simulink model "sampleModel2432_pp_1_1_difftest"  (R2018a)
settings: Solver=VariableStepAuto  StartTime=0.0  StopTime=10.0  RelTol=1e-3
undefined symbols (not defined in the file or in its folder): DiscIntNeverNeededParam, sigbuilder_block
libraries: simulink x293
(part 2 of 7)

== system sampleModel2432_pp_1_1_difftest/cfblk201 ==
  cfblk1 : Inport
  cfblk11 : Inport  Port=2
  Action Port : ActionPort  ActionType=then
  cfblk{3,7..8,10} (4 alike) : DiscreteZeroPole  Poles=[0 0.5]  Gain=1  SampleTime=-1
  cfblk14 : Delay
  cfblk4 : simulink/Discrete/Difference  ICPrevInput=0.0  OutMin=[]  OutMax=[]  OutDataTypeStr=Inherit: Inherit via back propagation  OutDataType=fixdt(1, 16)  OutScaling=2^-10  DoSatur=off
  cfblk5 : simulink/Continuous/PID Controller  Controller=PID  TimeDomain=Discrete-time  SampleTime=-1  IntegratorMethod=Forward Euler  FilterMethod=Forward Euler  Form=Parallel  UseFilter=on  ControllerParametersSource=internal  P=1  I=1  D=0  N=100  InitialConditionSource=internal  InitialConditionForIntegrator=0  InitialConditionForFilter=0  ExternalReset=none  LimitOutput=off  UpperSaturationLimit=inf  LowerSaturationLimit=-inf  LinearizeAsGain=off  AntiWindupMode=none  Kb=1  TrackingMode=off  Kt=1  PParamMin=[]  PParamMax=[]  IParamMin=[]  IParamMax=[]  DParamMin=[]  DParamMax=[]  NParamMin=[]  NParamMax=[]  KbParamMin=[]  KbParamMax=[]  KtParamMin=[]  KtParamMax=[]  POutMin=[]  POutMax=[]  IOutMin=[]  IOutMax=[]  DOutMin=[]  DOutMax=[]  NOutMin=[]  NOutMax=[]  KbOutMin=[]  KbOutMax=[]  KtOutMin=[]  KtOutMax=[]  IntegratorOutMin=[]  IntegratorOutMax=[]  FilterOutMin=[]  FilterOutMax=[]  SumOutMin=[]  SumOutMax=[]  SumI1OutMin=[]  SumI1OutMax=[]  SumI2OutMin=[]  SumI2OutMax=[]  SumI3OutMin=[]  SumI3OutMax=[]  SumDOutMin=[]  SumDOutMax=[]  SaturationOutMin=[]  SaturationOutMax=[]  IntegratorContinuousStateAttributes=''  IntegratorStateMustResolveToSignalObject=off  IntegratorRTWStateStorageClass=Auto  FilterContinuousStateAttributes=''  FilterStateMustResolveToSignalObject=off  FilterRTWStateStorageClass=Auto  DifferentiatorICPrevScaledInput=0  DifferentiatorOutMin=[]  DifferentiatorOutMax=[]  FilterDiffOutCoefMin=[]  FilterDiffOutCoefMax=[]  SumDenOutMin=[]  SumDenOutMax=[]  SumNumOutMin=[]  SumNumOutMax=[]  ReciprocalOutMin=[]  ReciprocalOutMax=[]  DivideOutMin=[]  DivideOutMax=[]  TunerSelectOption=Transfer Function Based (PID Tuner App)
  cfblk6 : Delay
  cfblk9 : DiscreteFir
  cyemi_{218..226} (9 alike) : DataTypeConversion  OutDataTypeStr=double
  cfblk2 : Outport
  cfblk12 : Outport  Port=2
  cfblk13 : Outport  Port=3
  wires:
  cfblk1/1 -> cfblk2/1
  cfblk10/1 -> cfblk13/1
  cfblk7/1 -> cfblk12/1
  cfblk4/1 -> cyemi_218/1, cyemi_225/1
  cyemi_218/1 -> cfblk10/1
  cyemi_219/1 -> cfblk14/1
  cfblk6/1 -> cyemi_219/1
  cyemi_220/1 -> cfblk3/1
  cfblk8/1 -> cyemi_220/1
  cyemi_221/1 -> cfblk4/1
  cfblk11/1 -> cyemi_221/1
  cyemi_222/1 -> cfblk5/1
  cfblk14/1 -> cyemi_222/1
  cyemi_223/1 -> cfblk6/1
  cfblk5/1 -> cyemi_223/1
  cyemi_224/1 -> cfblk7/1
  cfblk9/1 -> cyemi_224/1
  cyemi_225/1 -> cfblk8/1
  cyemi_226/1 -> cfblk9/1
  cfblk3/1 -> cyemi_226/1

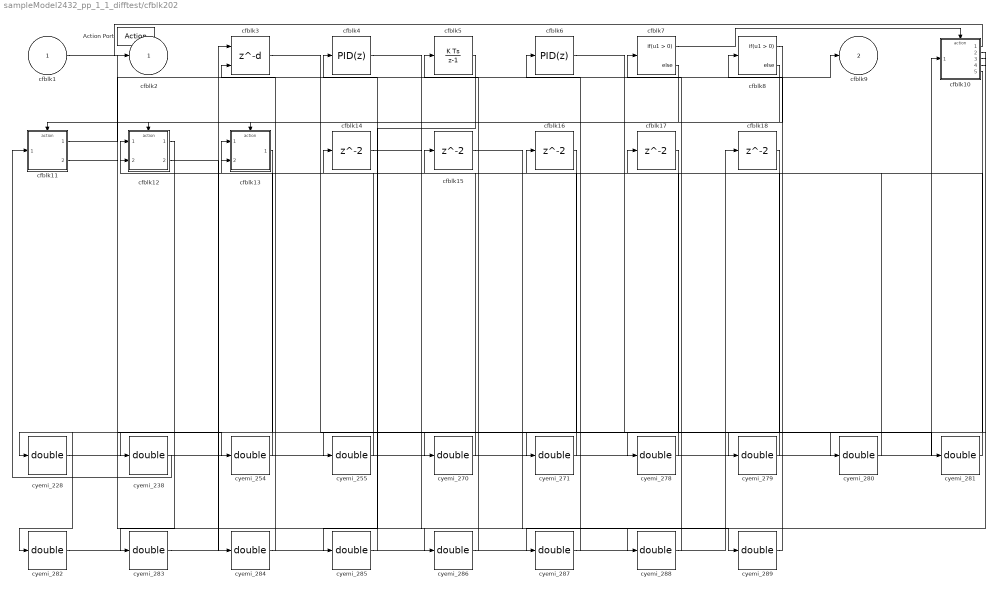
== system sampleModel2432_pp_1_1_difftest/cfblk202 ==
  cfblk1 : Inport
  Action Port : ActionPort  ActionType=else
  cfblk10 : Subsystem  TreatAsAtomicUnit=on
  cfblk11 : Subsystem  TreatAsAtomicUnit=on
  cfblk12 : Subsystem  TreatAsAtomicUnit=on
  cfblk13 : Subsystem  TreatAsAtomicUnit=on
  cfblk{14..18} (5 alike) : Delay
  cfblk3 : Delay  DelayLengthSource=Input port
      settings: InputPortMap=u0,p1
  cfblk4 : simulink/Continuous/PID Controller  Controller=PID  TimeDomain=Discrete-time  SampleTime=-1  IntegratorMethod=Forward Euler  FilterMethod=Forward Euler  Form=Parallel  UseFilter=on  ControllerParametersSource=internal  P=1  I=1  D=0  N=100  InitialConditionSource=internal  InitialConditionForIntegrator=0  InitialConditionForFilter=0  ExternalReset=none  LimitOutput=off  UpperSaturationLimit=inf  LowerSaturationLimit=-inf  LinearizeAsGain=off  AntiWindupMode=none  Kb=1  TrackingMode=off  Kt=1  PParamMin=[]  PParamMax=[]  IParamMin=[]  IParamMax=[]  DParamMin=[]  DParamMax=[]  NParamMin=[]  NParamMax=[]  KbParamMin=[]  KbParamMax=[]  KtParamMin=[]  KtParamMax=[]  POutMin=[]  POutMax=[]  IOutMin=[]  IOutMax=[]  DOutMin=[]  DOutMax=[]  NOutMin=[]  NOutMax=[]  KbOutMin=[]  KbOutMax=[]  KtOutMin=[]  KtOutMax=[]  IntegratorOutMin=[]  IntegratorOutMax=[]  FilterOutMin=[]  FilterOutMax=[]  SumOutMin=[]  SumOutMax=[]  SumI1OutMin=[]  SumI1OutMax=[]  SumI2OutMin=[]  SumI2OutMax=[]  SumI3OutMin=[]  SumI3OutMax=[]  SumDOutMin=[]  SumDOutMax=[]  SaturationOutMin=[]  SaturationOutMax=[]  IntegratorContinuousStateAttributes=''  IntegratorStateMustResolveToSignalObject=off  IntegratorRTWStateStorageClass=Auto  FilterContinuousStateAttributes=''  FilterStateMustResolveToSignalObject=off  FilterRTWStateStorageClass=Auto  DifferentiatorICPrevScaledInput=0  DifferentiatorOutMin=[]  DifferentiatorOutMax=[]  FilterDiffOutCoefMin=[]  FilterDiffOutCoefMax=[]  SumDenOutMin=[]  SumDenOutMax=[]  SumNumOutMin=[]  SumNumOutMax=[]  ReciprocalOutMin=[]  ReciprocalOutMax=[]  DivideOutMin=[]  DivideOutMax=[]  TunerSelectOption=Transfer Function Based (PID Tuner App)
  cfblk5 : DiscreteIntegrator  SampleTime=-1  ICPrevOutput=DiscIntNeverNeededParam  ICPrevScaledInput=DiscIntNeverNeededParam
  cfblk6 : simulink/Continuous/PID Controller  Controller=PID  TimeDomain=Discrete-time  SampleTime=-1  IntegratorMethod=Forward Euler  FilterMethod=Forward Euler  Form=Parallel  UseFilter=on  ControllerParametersSource=internal  P=1  I=1  D=0  N=100  InitialConditionSource=internal  InitialConditionForIntegrator=0  InitialConditionForFilter=0  ExternalReset=none  LimitOutput=off  UpperSaturationLimit=inf  LowerSaturationLimit=-inf  LinearizeAsGain=off  AntiWindupMode=none  Kb=1  TrackingMode=off  Kt=1  PParamMin=[]  PParamMax=[]  IParamMin=[]  IParamMax=[]  DParamMin=[]  DParamMax=[]  NParamMin=[]  NParamMax=[]  KbParamMin=[]  KbParamMax=[]  KtParamMin=[]  KtParamMax=[]  POutMin=[]  POutMax=[]  IOutMin=[]  IOutMax=[]  DOutMin=[]  DOutMax=[]  NOutMin=[]  NOutMax=[]  KbOutMin=[]  KbOutMax=[]  KtOutMin=[]  KtOutMax=[]  IntegratorOutMin=[]  IntegratorOutMax=[]  FilterOutMin=[]  FilterOutMax=[]  SumOutMin=[]  SumOutMax=[]  SumI1OutMin=[]  SumI1OutMax=[]  SumI2OutMin=[]  SumI2OutMax=[]  SumI3OutMin=[]  SumI3OutMax=[]  SumDOutMin=[]  SumDOutMax=[]  SaturationOutMin=[]  SaturationOutMax=[]  IntegratorContinuousStateAttributes=''  IntegratorStateMustResolveToSignalObject=off  IntegratorRTWStateStorageClass=Auto  FilterContinuousStateAttributes=''  FilterStateMustResolveToSignalObject=off  FilterRTWStateStorageClass=Auto  DifferentiatorICPrevScaledInput=0  DifferentiatorOutMin=[]  DifferentiatorOutMax=[]  FilterDiffOutCoefMin=[]  FilterDiffOutCoefMax=[]  SumDenOutMin=[]  SumDenOutMax=[]  SumNumOutMin=[]  SumNumOutMax=[]  ReciprocalOutMin=[]  ReciprocalOutMax=[]  DivideOutMin=[]  DivideOutMax=[]  TunerSelectOption=Transfer Function Based (PID Tuner App)
  cfblk7 : If  SampleTime=1
  cfblk8 : If  SampleTime=1
  cyemi_{228,238,254..255,270..271,278..289} (18 alike) : DataTypeConversion  OutDataTypeStr=double
  cfblk2 : Outport
  cfblk9 : Outport  Port=2
  wires:
  cfblk10/1(cfblk2) -> cfblk2/1
  cfblk11/1(cfblk2) -> cfblk9/1
  cfblk7/1 -> cfblk10/Action
  cfblk7/2 -> cfblk11/Action
  cfblk8/1 -> cfblk12/Action
  cfblk8/2 -> cfblk13/Action
  cyemi_228/1 -> cfblk10/1(cfblk1)
  cfblk13/1(cfblk2) -> cyemi_228/1
  cyemi_238/1 -> cfblk11/1(cfblk1)
  cfblk10/4(cfblk11) -> cyemi_238/1
  cyemi_254/1 -> cfblk12/1(cfblk1)
  cfblk1/1 -> cyemi_254/1
  cyemi_255/1 -> cfblk12/2(cfblk15)
  cfblk17/1 -> cyemi_255/1
  cyemi_270/1 -> cfblk13/1(cfblk1)
  cfblk18/1 -> cyemi_270/1
  cyemi_271/1 -> cfblk13/2(cfblk7)
  cfblk16/1 -> cyemi_271/1
  cyemi_278/1 -> cfblk14/1
  cfblk3/1 -> cyemi_278/1
  cyemi_279/1 -> cfblk15/1
  cfblk10/2(cfblk9) -> cyemi_279/1
  cyemi_280/1 -> cfblk16/1
  cfblk4/1 -> cyemi_280/1
  cyemi_281/1 -> cfblk17/1
  cfblk6/1 -> cyemi_281/1
  cyemi_282/1 -> cfblk18/1
  cfblk10/5(cfblk12) -> cyemi_282/1
  cyemi_283/1 -> cfblk3/1
  cfblk12/1(cfblk2) -> cyemi_283/1
  cyemi_284/1 -> cfblk3/2
  cfblk12/2(cfblk16) -> cyemi_284/1
  cyemi_285/1 -> cfblk4/1
  cfblk5/1 -> cyemi_285/1
  cyemi_286/1 -> cfblk5/1
  cfblk11/2(cfblk13) -> cyemi_286/1
  cyemi_287/1 -> cfblk6/1
  cfblk10/3(cfblk10) -> cyemi_287/1
  cyemi_288/1 -> cfblk7/1
  cfblk15/1 -> cyemi_288/1
  cyemi_289/1 -> cfblk8/1
  cfblk14/1 -> cyemi_289/1

== system sampleModel2432_pp_1_1_difftest/cfblk203 ==
  cfblk1 : Inport
  cfblk13 : Inport  Port=2
  cfblk14 : Inport  Port=3
  Action Port : ActionPort  ActionType=then
  cfblk3 : simulink/Continuous/PID Controller (2DOF)  Controller=PID  TimeDomain=Discrete-time  SampleTime=-1  IntegratorMethod=Forward Euler  FilterMethod=Forward Euler  Form=Parallel  UseFilter=on  ControllerParametersSource=internal  P=1  I=1  D=0  N=100  b=1  c=1  InitialConditionSource=internal  InitialConditionForIntegrator=0  InitialConditionForFilter=0  ExternalReset=none  LimitOutput=off  UpperSaturationLimit=inf  LowerSaturationLimit=-inf  LinearizeAsGain=off  AntiWindupMode=none  Kb=1  TrackingMode=off  Kt=1  PParamMin=[]  PParamMax=[]  IParamMin=[]  IParamMax=[]  DParamMin=[]  DParamMax=[]  NParamMin=[]  NParamMax=[]  bParamMin=[]  bParamMax=[]  cParamMin=[]  cParamMax=[]  KbParamMin=[]  KbParamMax=[]  KtParamMin=[]  KtParamMax=[]  POutMin=[]  POutMax=[]  IOutMin=[]  IOutMax=[]  DOutMin=[]  DOutMax=[]  NOutMin=[]  NOutMax=[]  bOutMin=[]  bOutMax=[]  cOutMin=[]  cOutMax=[]  KbOutMin=[]  KbOutMax=[]  KtOutMin=[]  KtOutMax=[]  IntegratorOutMin=[]  IntegratorOutMax=[]  FilterOutMin=[]  FilterOutMax=[]  SumOutMin=[]  SumOutMax=[]  Sum1OutMin=[]  Sum1OutMax=[]  Sum2OutMin=[]  Sum2OutMax=[]  Sum3OutMin=[]  Sum3OutMax=[]  SumI1OutMin=[]  SumI1OutMax=[]  SumI2OutMin=[]  SumI2OutMax=[]  SumI3OutMin=[]  SumI3OutMax=[]  SumDOutMin=[]  SumDOutMax=[]  SaturationOutMin=[]  SaturationOutMax=[]  IntegratorContinuousStateAttributes=''  IntegratorStateMustResolveToSignalObject=off  IntegratorRTWStateStorageClass=Auto  FilterContinuousStateAttributes=''  FilterStateMustResolveToSignalObject=off  FilterRTWStateStorageClass=Auto  DifferentiatorICPrevScaledInput=0  DifferentiatorOutMin=[]  DifferentiatorOutMax=[]  FilterDiffOutCoefMin=[]  FilterDiffOutCoefMax=[]  SumDenOutMin=[]  SumDenOutMax=[]  SumNumOutMin=[]  SumNumOutMax=[]  ReciprocalOutMin=[]  ReciprocalOutMax=[]  DivideOutMin=[]  DivideOutMax=[]  TunerSelectOption=Transfer Function Based (PID Tuner App)
  cfblk5 : Delay  ShowEnablePort=on
      settings: InputPortMap=u0,e6
  cfblk8 : DiscreteZeroPole  Poles=[0 0.5]  Gain=1  SampleTime=-1
  cyemi_{293..304} (12 alike) : DataTypeConversion  OutDataTypeStr=double
  cfblk2 : Outport
  cfblk15 : Outport  Port=2
  cfblk16 : Outport  Port=3
  wires:
  cfblk3/1 -> cfblk2/1
  cfblk14/1 -> cyemi_297/1, cyemi_304/1
  cfblk1/1 -> cyemi_294/1
  cfblk8/1 -> cyemi_295/1
  cyemi_296/1 -> cfblk3/1
  cyemi_297/1 -> cfblk3/2
  cyemi_299/1 -> cfblk5/1
  cyemi_300/1 -> cfblk5/2
  cfblk13/1 -> cyemi_300/1
  cfblk5/1 -> cyemi_301/1
  cyemi_303/1 -> cfblk8/1
  cyemi_304/1 -> cyemi_298/1
  cyemi_295/1 -> cfblk15/1
  cyemi_294/1 -> cyemi_302/1
  cyemi_301/1 -> cfblk16/1
  cyemi_302/1 -> cyemi_303/1, cyemi_296/1
  cyemi_298/1 -> cyemi_293/1
  cyemi_293/1 -> cyemi_299/1

== system sampleModel2432_pp_1_1_difftest/cfblk204 ==
  cfblk1 : Inport
  cfblk9 : Inport  Port=2
  cfblk10 : Inport  Port=3
  Action Port : ActionPort  ActionType=else
  cfblk13 : Subsystem  TreatAsAtomicUnit=on
  cfblk14 : Subsystem  TreatAsAtomicUnit=on
  cfblk15 : Delay
  cfblk16 : Delay
  cfblk3 : Delay
  cfblk4 : simulink/Discrete/Transfer Fcn Real Zero  ZeroZ=0.75  ICPrevInput=0.0  DoSatur=off
      settings: SourceProductName=Simulink  SourceProductBaseCode=SL
  cfblk5 : DiscreteFilter
  cfblk6 : DiscreteZeroPole  Poles=[0 0.5]  Gain=1  SampleTime=-1
  cfblk7 : DiscreteZeroPole  Poles=[0 0.5]  Gain=1  SampleTime=-1
  cfblk8 : If  SampleTime=1
  cyemi_{308..309,318..319,326..333} (12 alike) : DataTypeConversion  OutDataTypeStr=double
  cfblk2 : Outport
  cfblk11 : Outport  Port=2
  cfblk12 : Outport  Port=3
  wires:
  cfblk14/3(cfblk11) -> cfblk11/1
  cfblk14/4(cfblk12) -> cfblk12/1
  cfblk13/2(cfblk12) -> cfblk2/1
  cfblk8/1 -> cfblk13/Action
  cfblk8/2 -> cfblk14/Action
  cyemi_308/1 -> cfblk13/1(cfblk1)
  cfblk4/1 -> cyemi_308/1
  cyemi_309/1 -> cfblk13/2(cfblk11)
  cfblk14/2(cfblk10) -> cyemi_309/1
  cyemi_318/1 -> cfblk14/1(cfblk1)
  cfblk1/1 -> cyemi_318/1
  cyemi_319/1 -> cfblk14/2(cfblk9)
  cfblk15/1 -> cyemi_319/1
  cyemi_326/1 -> cfblk15/1
  cfblk3/1 -> cyemi_326/1
  cyemi_327/1 -> cfblk16/1
  cfblk13/1(cfblk2) -> cyemi_327/1
  cyemi_328/1 -> cfblk3/1
  cfblk5/1 -> cyemi_328/1
  cyemi_329/1 -> cfblk4/1
  cfblk7/1 -> cyemi_329/1
  cyemi_330/1 -> cfblk5/1
  cfblk14/1(cfblk2) -> cyemi_330/1
  cyemi_331/1 -> cfblk6/1
  cfblk10/1 -> cyemi_331/1
  cyemi_332/1 -> cfblk7/1
  cfblk6/1 -> cyemi_332/1
  cyemi_333/1 -> cfblk8/1
  cfblk16/1 -> cyemi_333/1

== system sampleModel2432_pp_1_1_difftest/cfblk205 ==
  cfblk1 : Inport
  Action Port : ActionPort  ActionType=then
  cfblk3 : simulink/Continuous/PID Controller  Controller=PID  TimeDomain=Discrete-time  SampleTime=-1  IntegratorMethod=Forward Euler  FilterMethod=Forward Euler  Form=Parallel  UseFilter=on  ControllerParametersSource=internal  P=1  I=1  D=0  N=100  InitialConditionSource=internal  InitialConditionForIntegrator=0  InitialConditionForFilter=0  ExternalReset=none  LimitOutput=off  UpperSaturationLimit=inf  LowerSaturationLimit=-inf  LinearizeAsGain=off  AntiWindupMode=none  Kb=1  TrackingMode=off  Kt=1  PParamMin=[]  PParamMax=[]  IParamMin=[]  IParamMax=[]  DParamMin=[]  DParamMax=[]  NParamMin=[]  NParamMax=[]  KbParamMin=[]  KbParamMax=[]  KtParamMin=[]  KtParamMax=[]  POutMin=[]  POutMax=[]  IOutMin=[]  IOutMax=[]  DOutMin=[]  DOutMax=[]  NOutMin=[]  NOutMax=[]  KbOutMin=[]  KbOutMax=[]  KtOutMin=[]  KtOutMax=[]  IntegratorOutMin=[]  IntegratorOutMax=[]  FilterOutMin=[]  FilterOutMax=[]  SumOutMin=[]  SumOutMax=[]  SumI1OutMin=[]  SumI1OutMax=[]  SumI2OutMin=[]  SumI2OutMax=[]  SumI3OutMin=[]  SumI3OutMax=[]  SumDOutMin=[]  SumDOutMax=[]  SaturationOutMin=[]  SaturationOutMax=[]  IntegratorContinuousStateAttributes=''  IntegratorStateMustResolveToSignalObject=off  IntegratorRTWStateStorageClass=Auto  FilterContinuousStateAttributes=''  FilterStateMustResolveToSignalObject=off  FilterRTWStateStorageClass=Auto  DifferentiatorICPrevScaledInput=0  DifferentiatorOutMin=[]  DifferentiatorOutMax=[]  FilterDiffOutCoefMin=[]  FilterDiffOutCoefMax=[]  SumDenOutMin=[]  SumDenOutMax=[]  SumNumOutMin=[]  SumNumOutMax=[]  ReciprocalOutMin=[]  ReciprocalOutMax=[]  DivideOutMin=[]  DivideOutMax=[]  TunerSelectOption=Transfer Function Based (PID Tuner App)
  cfblk4 : DiscreteFilter
  cfblk5 : simulink/Discrete/Transfer Fcn Real Zero  ZeroZ=0.75  ICPrevInput=0.0  DoSatur=off
      settings: SourceProductName=Simulink  SourceProductBaseCode=SL
  cfblk6 : simulink/Discrete/Transfer Fcn Real Zero  ZeroZ=0.75  ICPrevInput=0.0  DoSatur=off
      settings: SourceProductName=Simulink  SourceProductBaseCode=SL
  cyemi_{335..338} (4 alike) : DataTypeConversion  OutDataTypeStr=double
  cfblk2 : Outport
  cfblk7 : Outport  Port=2
  cfblk8 : Outport  Port=3
  wires:
  cfblk5/1 -> cyemi_335/1, cyemi_338/1
  cfblk3/1 -> cfblk2/1
  cfblk4/1 -> cfblk7/1, cfblk8/1
  cyemi_335/1 -> cfblk3/1
  cyemi_336/1 -> cfblk4/1
  cfblk6/1 -> cyemi_336/1
  cyemi_337/1 -> cfblk5/1
  cfblk1/1 -> cyemi_337/1
  cyemi_338/1 -> cfblk6/1

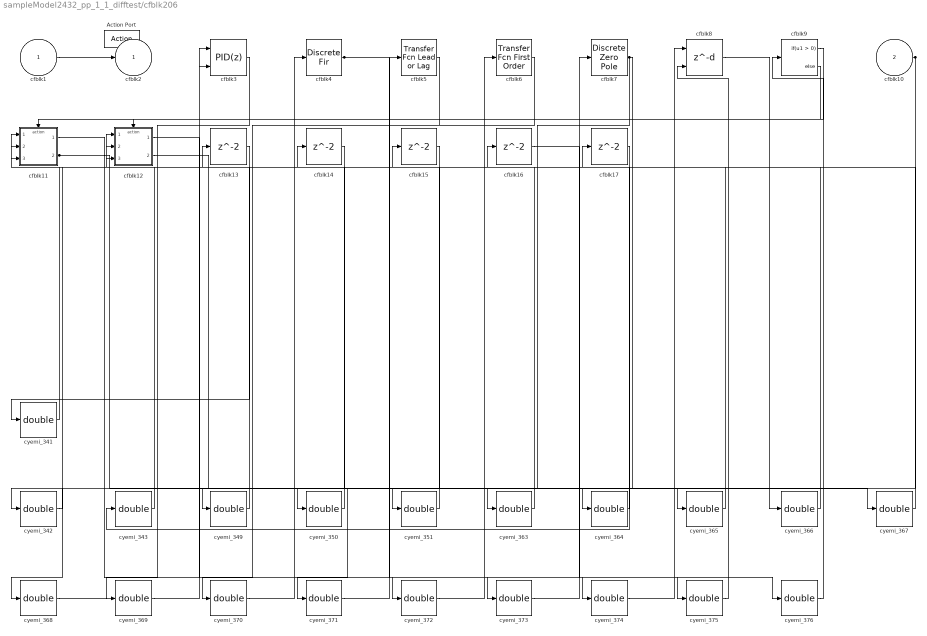
== system sampleModel2432_pp_1_1_difftest/cfblk206 ==
  cfblk1 : Inport
  cfblk10 : Inport  Port=2
  Action Port : ActionPort  ActionType=else
  cfblk11 : Subsystem  TreatAsAtomicUnit=on
  cfblk12 : Subsystem  TreatAsAtomicUnit=on
  cfblk{13..17} (5 alike) : Delay
  cfblk3 : simulink/Continuous/PID Controller (2DOF)  Controller=PID  TimeDomain=Discrete-time  SampleTime=-1  IntegratorMethod=Forward Euler  FilterMethod=Forward Euler  Form=Parallel  UseFilter=on  ControllerParametersSource=internal  P=1  I=1  D=0  N=100  b=1  c=1  InitialConditionSource=internal  InitialConditionForIntegrator=0  InitialConditionForFilter=0  ExternalReset=none  LimitOutput=off  UpperSaturationLimit=inf  LowerSaturationLimit=-inf  LinearizeAsGain=off  AntiWindupMode=none  Kb=1  TrackingMode=off  Kt=1  PParamMin=[]  PParamMax=[]  IParamMin=[]  IParamMax=[]  DParamMin=[]  DParamMax=[]  NParamMin=[]  NParamMax=[]  bParamMin=[]  bParamMax=[]  cParamMin=[]  cParamMax=[]  KbParamMin=[]  KbParamMax=[]  KtParamMin=[]  KtParamMax=[]  POutMin=[]  POutMax=[]  IOutMin=[]  IOutMax=[]  DOutMin=[]  DOutMax=[]  NOutMin=[]  NOutMax=[]  bOutMin=[]  bOutMax=[]  cOutMin=[]  cOutMax=[]  KbOutMin=[]  KbOutMax=[]  KtOutMin=[]  KtOutMax=[]  IntegratorOutMin=[]  IntegratorOutMax=[]  FilterOutMin=[]  FilterOutMax=[]  SumOutMin=[]  SumOutMax=[]  Sum1OutMin=[]  Sum1OutMax=[]  Sum2OutMin=[]  Sum2OutMax=[]  Sum3OutMin=[]  Sum3OutMax=[]  SumI1OutMin=[]  SumI1OutMax=[]  SumI2OutMin=[]  SumI2OutMax=[]  SumI3OutMin=[]  SumI3OutMax=[]  SumDOutMin=[]  SumDOutMax=[]  SaturationOutMin=[]  SaturationOutMax=[]  IntegratorContinuousStateAttributes=''  IntegratorStateMustResolveToSignalObject=off  IntegratorRTWStateStorageClass=Auto  FilterContinuousStateAttributes=''  FilterStateMustResolveToSignalObject=off  FilterRTWStateStorageClass=Auto  DifferentiatorICPrevScaledInput=0  DifferentiatorOutMin=[]  DifferentiatorOutMax=[]  FilterDiffOutCoefMin=[]  FilterDiffOutCoefMax=[]  SumDenOutMin=[]  SumDenOutMax=[]  SumNumOutMin=[]  SumNumOutMax=[]  ReciprocalOutMin=[]  ReciprocalOutMax=[]  DivideOutMin=[]  DivideOutMax=[]  TunerSelectOption=Transfer Function Based (PID Tuner App)
  cfblk4 : DiscreteFir
  cfblk5 : simulink/Discrete/Transfer Fcn Lead or Lag  PoleZ=0.95  ZeroZ=0.75  ICPrevOutput=0.0  ICPrevInput=0.0  DoSatur=off
      settings: SourceProductName=Simulink  SourceProductBaseCode=SL
  cfblk6 : simulink/Discrete/Transfer Fcn First Order  PoleZ=0.95  ICPrevOutput=0.0  DoSatur=off
      settings: SourceProductName=Simulink
  cfblk7 : DiscreteZeroPole  Poles=[0 0.5]  Gain=1  SampleTime=-1
  cfblk8 : Delay  DelayLengthSource=Input port
      settings: InputPortMap=u0,p1
  cfblk9 : If  SampleTime=1
  cyemi_{341..343,349..351,363..376} (20 alike) : DataTypeConversion  OutDataTypeStr=double
  cfblk2 : Outport
  wires:
  cfblk4/1 -> cyemi_365/1, cyemi_373/1
  cfblk1/1 -> cfblk2/1
  cfblk10/1 -> cyemi_368/1, cyemi_371/1
  cfblk7/1 -> cyemi_363/1, cyemi_364/1
  cfblk11/2(cfblk10) -> cyemi_350/1, cyemi_374/1
  cfblk9/1 -> cfblk11/Action
  cfblk9/2 -> cfblk12/Action
  cyemi_341/1 -> cfblk11/1(cfblk1)
  cfblk13/1 -> cyemi_341/1
  cyemi_342/1 -> cfblk11/2(cfblk8)
  cfblk3/1 -> cyemi_342/1
  cyemi_343/1 -> cfblk11/3(cfblk9)
  cfblk17/1 -> cyemi_343/1
  cyemi_349/1 -> cfblk12/1(cfblk1)
  cfblk5/1 -> cyemi_349/1
  cyemi_350/1 -> cfblk12/2(cfblk13)
  cyemi_351/1 -> cfblk12/3(cfblk14)
  cfblk15/1 -> cyemi_351/1
  cyemi_363/1 -> cfblk13/1
  cyemi_364/1 -> cfblk14/1
  cyemi_365/1 -> cfblk15/1
  cyemi_366/1 -> cfblk16/1
  cfblk8/1 -> cyemi_366/1
  cyemi_367/1 -> cfblk17/1
  cfblk12/2(cfblk15) -> cyemi_367/1
  cyemi_368/1 -> cfblk3/1
  cyemi_369/1 -> cfblk3/2
  cfblk14/1 -> cyemi_369/1
  cyemi_370/1 -> cfblk4/1
  cfblk6/1 -> cyemi_370/1
  cyemi_371/1 -> cfblk5/1
  cyemi_372/1 -> cfblk6/1
  cfblk11/1(cfblk2) -> cyemi_372/1
  cyemi_373/1 -> cfblk7/1
  cyemi_374/1 -> cfblk8/1
  cyemi_375/1 -> cfblk8/2
  cfblk12/1(cfblk2) -> cyemi_375/1
  cyemi_376/1 -> cfblk9/1
  cfblk16/1 -> cyemi_376/1

== system sampleModel2432_pp_1_1_difftest/cfblk207 ==
  cfblk1 : Inport
  cfblk8 : Inport  Port=2
  Action Port : ActionPort  ActionType=then
  cfblk10 : Delay
  cfblk4 : simulink/Discrete/Transfer Fcn Lead or Lag  PoleZ=0.95  ZeroZ=0.75  ICPrevOutput=0.0  ICPrevInput=0.0  DoSatur=off
      settings: SourceProductName=Simulink  SourceProductBaseCode=SL
  cfblk5 : DiscreteFir
  cfblk6 : Delay
  cfblk7 : Delay  ShowEnablePort=on
      settings: InputPortMap=u0,e6
  cyemi_{379..385} (7 alike) : DataTypeConversion  OutDataTypeStr=double
  cfblk2 : Outport
  cfblk9 : Outport  Port=2
  wires:
  cfblk1/1 -> cfblk9/1
  cyemi_379/1 -> cfblk10/1
  cfblk6/1 -> cyemi_379/1
  cfblk8/1 -> cyemi_380/1
  cyemi_381/1 -> cfblk4/1
  cfblk5/1 -> cyemi_381/1
  cyemi_382/1 -> cfblk5/1
  cyemi_383/1 -> cfblk6/1
  cfblk7/1 -> cyemi_383/1
  cyemi_384/1 -> cfblk7/1
  cfblk10/1 -> cyemi_384/1
  cyemi_385/1 -> cfblk7/2
  cfblk4/1 -> cyemi_385/1
  cyemi_380/1 -> cyemi_382/1, cfblk2/1

== system sampleModel2432_pp_1_1_difftest/cfblk208 ==
  cfblk1 : Inport
  Action Port : ActionPort  ActionType=else
  cfblk3 : Delay  ShowEnablePort=on
      settings: InputPortMap=u0,e6
  cfblk4 : DiscreteTransferFcn
  cfblk5 : simulink/Continuous/PID Controller  Controller=PID  TimeDomain=Discrete-time  SampleTime=-1  IntegratorMethod=Forward Euler  FilterMethod=Forward Euler  Form=Parallel  UseFilter=on  ControllerParametersSource=internal  P=1  I=1  D=0  N=100  InitialConditionSource=internal  InitialConditionForIntegrator=0  InitialConditionForFilter=0  ExternalReset=none  LimitOutput=off  UpperSaturationLimit=inf  LowerSaturationLimit=-inf  LinearizeAsGain=off  AntiWindupMode=none  Kb=1  TrackingMode=off  Kt=1  PParamMin=[]  PParamMax=[]  IParamMin=[]  IParamMax=[]  DParamMin=[]  DParamMax=[]  NParamMin=[]  NParamMax=[]  KbParamMin=[]  KbParamMax=[]  KtParamMin=[]  KtParamMax=[]  POutMin=[]  POutMax=[]  IOutMin=[]  IOutMax=[]  DOutMin=[]  DOutMax=[]  NOutMin=[]  NOutMax=[]  KbOutMin=[]  KbOutMax=[]  KtOutMin=[]  KtOutMax=[]  IntegratorOutMin=[]  IntegratorOutMax=[]  FilterOutMin=[]  FilterOutMax=[]  SumOutMin=[]  SumOutMax=[]  SumI1OutMin=[]  SumI1OutMax=[]  SumI2OutMin=[]  SumI2OutMax=[]  SumI3OutMin=[]  SumI3OutMax=[]  SumDOutMin=[]  SumDOutMax=[]  SaturationOutMin=[]  SaturationOutMax=[]  IntegratorContinuousStateAttributes=''  IntegratorStateMustResolveToSignalObject=off  IntegratorRTWStateStorageClass=Auto  FilterContinuousStateAttributes=''  FilterStateMustResolveToSignalObject=off  FilterRTWStateStorageClass=Auto  DifferentiatorICPrevScaledInput=0  DifferentiatorOutMin=[]  DifferentiatorOutMax=[]  FilterDiffOutCoefMin=[]  FilterDiffOutCoefMax=[]  SumDenOutMin=[]  SumDenOutMax=[]  SumNumOutMin=[]  SumNumOutMax=[]  ReciprocalOutMin=[]  ReciprocalOutMax=[]  DivideOutMin=[]  DivideOutMax=[]  TunerSelectOption=Transfer Function Based (PID Tuner App)
  cfblk6 : DiscreteFilter
  cfblk9 : Delay
  cyemi_{387..392} (6 alike) : DataTypeConversion  OutDataTypeStr=double
  cfblk2 : Outport
  cfblk7 : Outport  Port=2
  cfblk8 : Outport  Port=3
  wires:
  cfblk6/1 -> cfblk8/1
  cfblk4/1 -> cfblk7/1, cyemi_391/1
  cfblk5/1 -> cfblk2/1, cyemi_389/1, cyemi_392/1
  cyemi_387/1 -> cfblk3/1
  cfblk1/1 -> cyemi_387/1
  cyemi_388/1 -> cfblk3/2
  cfblk9/1 -> cyemi_388/1
  cyemi_389/1 -> cfblk4/1
  cyemi_390/1 -> cfblk5/1
  cfblk3/1 -> cyemi_390/1
  cyemi_391/1 -> cfblk6/1
  cyemi_392/1 -> cfblk9/1

== system sampleModel2432_pp_1_1_difftest/cfblk209 ==
  cfblk1 : Inport
  Action Port : ActionPort  ActionType=then
  cfblk3 : simulink/Discrete/Difference  ICPrevInput=0.0  OutMin=[]  OutMax=[]  OutDataTypeStr=Inherit: Inherit via back propagation  OutDataType=fixdt(1, 16)  OutScaling=2^-10  DoSatur=off
  cyemi_394 : DataTypeConversion  OutDataTypeStr=double
  cfblk2 : Outport
  cfblk4 : Outport  Port=2
  cfblk5 : Outport  Port=3
  cfblk6 : Outport  Port=4
  cfblk7 : Outport  Port=5
  wires:
  cfblk1/1 -> cfblk6/1, cfblk7/1, cyemi_394/1
  cfblk3/1 -> cfblk4/1, cfblk2/1, cfblk5/1
  cyemi_394/1 -> cfblk3/1

== system sampleModel2432_pp_1_1_difftest/cfblk210 ==
  cfblk1 : Inport
  Action Port : ActionPort  ActionType=else
  cfblk10 : Subsystem  TreatAsAtomicUnit=on
  cfblk11 : Subsystem  TreatAsAtomicUnit=on
  cfblk{12..15} (4 alike) : Delay
  cfblk3 : simulink/Discrete/Difference  ICPrevInput=0.0  OutMin=[]  OutMax=[]  OutDataTypeStr=Inherit: Inherit via back propagation  OutDataType=fixdt(1, 16)  OutScaling=2^-10  DoSatur=off
  cfblk4 : DiscreteFir
  cfblk5 : simulink/Discrete/Transfer Fcn Real Zero  ZeroZ=0.75  ICPrevInput=0.0  DoSatur=off
      settings: SourceProductName=Simulink  SourceProductBaseCode=SL
  cfblk6 : DiscreteStateSpace  SampleTime=-1
  cfblk7 : DiscreteIntegrator  SampleTime=-1  ICPrevOutput=DiscIntNeverNeededParam  ICPrevScaledInput=DiscIntNeverNeededParam
  cfblk8 : Delay  ShowEnablePort=on
      settings: InputPortMap=u0,e6
  cfblk9 : If  SampleTime=1
  cyemi_{398,405..406,420..431} (15 alike) : DataTypeConversion  OutDataTypeStr=double
  cfblk2 : Outport
  wires:
  cfblk11/3(cfblk14) -> cfblk2/1
  cfblk9/1 -> cfblk10/Action
  cfblk9/2 -> cfblk11/Action
  cyemi_398/1 -> cfblk10/1(cfblk1)
  cfblk13/1 -> cyemi_398/1
  cyemi_405/1 -> cfblk11/1(cfblk1)
  cfblk3/1 -> cyemi_405/1
  cyemi_406/1 -> cfblk11/2(cfblk12)
  cfblk15/1 -> cyemi_406/1
  cyemi_420/1 -> cfblk12/1
  cfblk10/1(cfblk2) -> cyemi_420/1
  cyemi_421/1 -> cfblk13/1
  cfblk5/1 -> cyemi_421/1
  cyemi_422/1 -> cfblk14/1
  cfblk8/1 -> cyemi_422/1
  cyemi_423/1 -> cfblk15/1
  cfblk7/1 -> cyemi_423/1
  cyemi_424/1 -> cfblk3/1
  cfblk1/1 -> cyemi_424/1
  cyemi_425/1 -> cfblk4/1
  cfblk6/1 -> cyemi_425/1
  cyemi_426/1 -> cfblk5/1
  cfblk10/2(cfblk7) -> cyemi_426/1
  cyemi_427/1 -> cfblk6/1
  cfblk11/1(cfblk2) -> cyemi_427/1
  cyemi_428/1 -> cfblk7/1
  cfblk11/2(cfblk13) -> cyemi_428/1
  cyemi_429/1 -> cfblk8/1
  cfblk12/1 -> cyemi_429/1
  cyemi_430/1 -> cfblk8/2
  cfblk4/1 -> cyemi_430/1
  cyemi_431/1 -> cfblk9/1
  cfblk14/1 -> cyemi_431/1

== system sampleModel2432_pp_1_1_difftest/cfblk211 ==
  cfblk1 : Inport
  cfblk7 : Inport  Port=2
  Action Port : ActionPort  ActionType=then
  cfblk5 : simulink/Discrete/Transfer Fcn Real Zero  ZeroZ=0.75  ICPrevInput=0.0  DoSatur=off
      settings: SourceProductName=Simulink  SourceProductBaseCode=SL
  cyemi_{434..437} (4 alike) : DataTypeConversion  OutDataTypeStr=double
  cfblk2 : Outport
  wires:
  cfblk5/1 -> cyemi_435/1
  cyemi_436/1 -> cfblk5/1
  cfblk7/1 -> cyemi_436/1
  cfblk1/1 -> cyemi_437/1
  cyemi_434/1 -> cfblk2/1
  cyemi_435/1 -> cyemi_434/1

== system sampleModel2432_pp_1_1_difftest/cfblk212 ==
  cfblk1 : Inport
  cfblk9 : Inport  Port=2
  Action Port : ActionPort  ActionType=else
  cfblk3 : DiscreteZeroPole  Poles=[0 0.5]  Gain=1  SampleTime=-1
  cfblk4 : DiscreteTransferFcn
  cfblk5 : DiscreteFilter
  cfblk6 : simulink/Discrete/Transfer Fcn Real Zero  ZeroZ=0.75  ICPrevInput=0.0  DoSatur=off
      settings: SourceProductName=Simulink  SourceProductBaseCode=SL
  cfblk7 : DiscreteIntegrator  SampleTime=-1  ICPrevOutput=DiscIntNeverNeededParam  ICPrevScaledInput=DiscIntNeverNeededParam
  cfblk8 : simulink/Discrete/Transfer Fcn First Order  PoleZ=0.95  ICPrevOutput=0.0  DoSatur=off
      settings: SourceProductName=Simulink
  cyemi_{440..445} (6 alike) : DataTypeConversion  OutDataTypeStr=double
  cfblk2 : Outport
  cfblk10 : Outport  Port=2
  cfblk11 : Outport  Port=3
  cfblk12 : Outport  Port=4
  wires:
  cfblk7/1 -> cfblk12/1, cyemi_441/1
  cfblk5/1 -> cfblk10/1, cyemi_443/1
  cfblk3/1 -> cfblk11/1
  cfblk4/1 -> cfblk2/1
  cyemi_440/1 -> cfblk3/1
  cfblk8/1 -> cyemi_440/1
  cyemi_441/1 -> cfblk4/1
  cyemi_442/1 -> cfblk5/1
  cfblk9/1 -> cyemi_442/1
  cyemi_443/1 -> cfblk6/1
  cyemi_444/1 -> cfblk7/1
  cfblk1/1 -> cyemi_444/1
  cyemi_445/1 -> cfblk8/1
  cfblk6/1 -> cyemi_445/1

== system sampleModel2432_pp_1_1_difftest/cfblk213 ==
  cfblk1 : Inport
  cfblk7 : Inport  Port=2
  cfblk8 : Inport  Port=3
  Action Port : ActionPort  ActionType=then
  cfblk3 : Delay
  cfblk5 : DiscreteIntegrator  SampleTime=-1  ICPrevOutput=DiscIntNeverNeededParam  ICPrevScaledInput=DiscIntNeverNeededParam
  cfblk6 : DiscreteZeroPole  Poles=[0 0.5]  Gain=1  SampleTime=-1
  cyemi_{449..452} (4 alike) : DataTypeConversion  OutDataTypeStr=double
  cfblk2 : Outport
  cfblk9 : Outport  Port=2
  wires:
  cfblk5/1 -> cfblk9/1
  cfblk3/1 -> cfblk2/1
  cyemi_449/1 -> cfblk3/1
  cfblk7/1 -> cyemi_450/1
  cyemi_451/1 -> cfblk5/1
  cfblk8/1 -> cyemi_451/1
  cyemi_452/1 -> cfblk6/1
  cfblk1/1 -> cyemi_452/1
  cyemi_450/1 -> cyemi_449/1

== system sampleModel2432_pp_1_1_difftest/cfblk214 ==
  cfblk1 : Inport
  cfblk9 : Inport  Port=2
  Action Port : ActionPort  ActionType=else
  cfblk10 : Delay
  cfblk3 : simulink/Discrete/Tapped Delay  vinit=0.0  samptime=-1  NumDelays=1  DelayOrder=Oldest  includeCurrent=off
  cfblk4 : simulink/Discrete/Tapped Delay  vinit=0.0  samptime=-1  NumDelays=1  DelayOrder=Oldest  includeCurrent=off
  cfblk5 : DiscreteFilter
  cfblk6 : simulink/Discrete/Transfer Fcn Real Zero  ZeroZ=0.75  ICPrevInput=0.0  DoSatur=off
      settings: SourceProductName=Simulink  SourceProductBaseCode=SL
  cfblk7 : DiscreteIntegrator  SampleTime=-1  ICPrevOutput=DiscIntNeverNeededParam  ICPrevScaledInput=DiscIntNeverNeededParam
  cfblk8 : simulink/Continuous/PID Controller  Controller=PID  TimeDomain=Discrete-time  SampleTime=-1  IntegratorMethod=Forward Euler  FilterMethod=Forward Euler  Form=Parallel  UseFilter=on  ControllerParametersSource=internal  P=1  I=1  D=0  N=100  InitialConditionSource=internal  InitialConditionForIntegrator=0  InitialConditionForFilter=0  ExternalReset=none  LimitOutput=off  UpperSaturationLimit=inf  LowerSaturationLimit=-inf  LinearizeAsGain=off  AntiWindupMode=none  Kb=1  TrackingMode=off  Kt=1  PParamMin=[]  PParamMax=[]  IParamMin=[]  IParamMax=[]  DParamMin=[]  DParamMax=[]  NParamMin=[]  NParamMax=[]  KbParamMin=[]  KbParamMax=[]  KtParamMin=[]  KtParamMax=[]  POutMin=[]  POutMax=[]  IOutMin=[]  IOutMax=[]  DOutMin=[]  DOutMax=[]  NOutMin=[]  NOutMax=[]  KbOutMin=[]  KbOutMax=[]  KtOutMin=[]  KtOutMax=[]  IntegratorOutMin=[]  IntegratorOutMax=[]  FilterOutMin=[]  FilterOutMax=[]  SumOutMin=[]  SumOutMax=[]  SumI1OutMin=[]  SumI1OutMax=[]  SumI2OutMin=[]  SumI2OutMax=[]  SumI3OutMin=[]  SumI3OutMax=[]  SumDOutMin=[]  SumDOutMax=[]  SaturationOutMin=[]  SaturationOutMax=[]  IntegratorContinuousStateAttributes=''  IntegratorStateMustResolveToSignalObject=off  IntegratorRTWStateStorageClass=Auto  FilterContinuousStateAttributes=''  FilterStateMustResolveToSignalObject=off  FilterRTWStateStorageClass=Auto  DifferentiatorICPrevScaledInput=0  DifferentiatorOutMin=[]  DifferentiatorOutMax=[]  FilterDiffOutCoefMin=[]  FilterDiffOutCoefMax=[]  SumDenOutMin=[]  SumDenOutMax=[]  SumNumOutMin=[]  SumNumOutMax=[]  ReciprocalOutMin=[]  ReciprocalOutMax=[]  DivideOutMin=[]  DivideOutMax=[]  TunerSelectOption=Transfer Function Based (PID Tuner App)
  cyemi_{455..461} (7 alike) : DataTypeConversion  OutDataTypeStr=double
  cfblk2 : Outport
  wires:
  cfblk3/1 -> cfblk2/1
  cyemi_455/1 -> cfblk10/1
  cfblk8/1 -> cyemi_455/1
  cyemi_456/1 -> cfblk3/1
  cfblk6/1 -> cyemi_456/1
  cyemi_457/1 -> cfblk4/1
  cfblk10/1 -> cyemi_457/1
  cyemi_458/1 -> cfblk5/1
  cfblk9/1 -> cyemi_458/1
  cyemi_459/1 -> cfblk6/1
  cfblk1/1 -> cyemi_459/1
  cyemi_460/1 -> cfblk7/1
  cfblk5/1 -> cyemi_460/1
  cyemi_461/1 -> cfblk8/1
  cfblk4/1 -> cyemi_461/1

== system sampleModel2432_pp_1_1_difftest/cfblk215 ==
  cfblk1 : Inport
  cfblk10 : Inport  Port=2
  Action Port : ActionPort  ActionType=then
  cfblk13 : Delay
  cfblk3 : simulink/Discrete/Difference  ICPrevInput=0.0  OutMin=[]  OutMax=[]  OutDataTypeStr=Inherit: Inherit via back propagation  OutDataType=fixdt(1, 16)  OutScaling=2^-10  DoSatur=off
  cfblk4 : simulink/Continuous/PID Controller  Controller=PID  TimeDomain=Discrete-time  SampleTime=-1  IntegratorMethod=Forward Euler  FilterMethod=Forward Euler  Form=Parallel  UseFilter=on  ControllerParametersSource=internal  P=1  I=1  D=0  N=100  InitialConditionSource=internal  InitialConditionForIntegrator=0  InitialConditionForFilter=0  ExternalReset=none  LimitOutput=off  UpperSaturationLimit=inf  LowerSaturationLimit=-inf  LinearizeAsGain=off  AntiWindupMode=none  Kb=1  TrackingMode=off  Kt=1  PParamMin=[]  PParamMax=[]  IParamMin=[]  IParamMax=[]  DParamMin=[]  DParamMax=[]  NParamMin=[]  NParamMax=[]  KbParamMin=[]  KbParamMax=[]  KtParamMin=[]  KtParamMax=[]  POutMin=[]  POutMax=[]  IOutMin=[]  IOutMax=[]  DOutMin=[]  DOutMax=[]  NOutMin=[]  NOutMax=[]  KbOutMin=[]  KbOutMax=[]  KtOutMin=[]  KtOutMax=[]  IntegratorOutMin=[]  IntegratorOutMax=[]  FilterOutMin=[]  FilterOutMax=[]  SumOutMin=[]  SumOutMax=[]  SumI1OutMin=[]  SumI1OutMax=[]  SumI2OutMin=[]  SumI2OutMax=[]  SumI3OutMin=[]  SumI3OutMax=[]  SumDOutMin=[]  SumDOutMax=[]  SaturationOutMin=[]  SaturationOutMax=[]  IntegratorContinuousStateAttributes=''  IntegratorStateMustResolveToSignalObject=off  IntegratorRTWStateStorageClass=Auto  FilterContinuousStateAttributes=''  FilterStateMustResolveToSignalObject=off  FilterRTWStateStorageClass=Auto  DifferentiatorICPrevScaledInput=0  DifferentiatorOutMin=[]  DifferentiatorOutMax=[]  FilterDiffOutCoefMin=[]  FilterDiffOutCoefMax=[]  SumDenOutMin=[]  SumDenOutMax=[]  SumNumOutMin=[]  SumNumOutMax=[]  ReciprocalOutMin=[]  ReciprocalOutMax=[]  DivideOutMin=[]  DivideOutMax=[]  TunerSelectOption=Transfer Function Based (PID Tuner App)
  cfblk5 : simulink/Discrete/Difference  ICPrevInput=0.0  OutMin=[]  OutMax=[]  OutDataTypeStr=Inherit: Inherit via back propagation  OutDataType=fixdt(1, 16)  OutScaling=2^-10  DoSatur=off
  cfblk6 : Delay  DelayLengthSource=Input port
      settings: InputPortMap=u0,p1
  cfblk7 : Delay  DelayLengthSource=Input port
      settings: InputPortMap=u0,p1
  cfblk8 : simulink/Discrete/Transfer Fcn Lead or Lag  PoleZ=0.95  ZeroZ=0.75  ICPrevOutput=0.0  ICPrevInput=0.0  DoSatur=off
      settings: SourceProductName=Simulink  SourceProductBaseCode=SL
  cfblk9 : DiscreteFilter
  cyemi_{464..473} (10 alike) : DataTypeConversion  OutDataTypeStr=double
  cfblk2 : Outport
  cfblk11 : Outport  Port=2
  cfblk12 : Outport  Port=3
  wires:
  cfblk3/1 -> cyemi_469/1, cyemi_470/1
  cfblk1/1 -> cfblk12/1
  cfblk9/1 -> cfblk2/1
  cfblk7/1 -> cfblk11/1, cyemi_467/1, cyemi_473/1
  cyemi_464/1 -> cfblk13/1
  cfblk4/1 -> cyemi_464/1
  cyemi_465/1 -> cfblk3/1
  cfblk13/1 -> cyemi_465/1
  cyemi_466/1 -> cfblk4/1
  cfblk6/1 -> cyemi_466/1
  cyemi_467/1 -> cfblk5/1
  cyemi_468/1 -> cfblk6/1
  cfblk8/1 -> cyemi_468/1
  cyemi_469/1 -> cfblk6/2
  cyemi_470/1 -> cfblk7/1
  cyemi_471/1 -> cfblk7/2
  cfblk10/1 -> cyemi_471/1
  cyemi_472/1 -> cfblk8/1
  cfblk5/1 -> cyemi_472/1
  cyemi_473/1 -> cfblk9/1

== system sampleModel2432_pp_1_1_difftest/cfblk216 ==
  cfblk1 : Inport
  cfblk13 : Inport  Port=2
  Action Port : ActionPort  ActionType=else
  cfblk6 : simulink/Continuous/PID Controller (2DOF)  Controller=PID  TimeDomain=Discrete-time  SampleTime=-1  IntegratorMethod=Forward Euler  FilterMethod=Forward Euler  Form=Parallel  UseFilter=on  ControllerParametersSource=internal  P=1  I=1  D=0  N=100  b=1  c=1  InitialConditionSource=internal  InitialConditionForIntegrator=0  InitialConditionForFilter=0  ExternalReset=none  LimitOutput=off  UpperSaturationLimit=inf  LowerSaturationLimit=-inf  LinearizeAsGain=off  AntiWindupMode=none  Kb=1  TrackingMode=off  Kt=1  PParamMin=[]  PParamMax=[]  IParamMin=[]  IParamMax=[]  DParamMin=[]  DParamMax=[]  NParamMin=[]  NParamMax=[]  bParamMin=[]  bParamMax=[]  cParamMin=[]  cParamMax=[]  KbParamMin=[]  KbParamMax=[]  KtParamMin=[]  KtParamMax=[]  POutMin=[]  POutMax=[]  IOutMin=[]  IOutMax=[]  DOutMin=[]  DOutMax=[]  NOutMin=[]  NOutMax=[]  bOutMin=[]  bOutMax=[]  cOutMin=[]  cOutMax=[]  KbOutMin=[]  KbOutMax=[]  KtOutMin=[]  KtOutMax=[]  IntegratorOutMin=[]  IntegratorOutMax=[]  FilterOutMin=[]  FilterOutMax=[]  SumOutMin=[]  SumOutMax=[]  Sum1OutMin=[]  Sum1OutMax=[]  Sum2OutMin=[]  Sum2OutMax=[]  Sum3OutMin=[]  Sum3OutMax=[]  SumI1OutMin=[]  SumI1OutMax=[]  SumI2OutMin=[]  SumI2OutMax=[]  SumI3OutMin=[]  SumI3OutMax=[]  SumDOutMin=[]  SumDOutMax=[]  SaturationOutMin=[]  SaturationOutMax=[]  IntegratorContinuousStateAttributes=''  IntegratorStateMustResolveToSignalObject=off  IntegratorRTWStateStorageClass=Auto  FilterContinuousStateAttributes=''  FilterStateMustResolveToSignalObject=off  FilterRTWStateStorageClass=Auto  DifferentiatorICPrevScaledInput=0  DifferentiatorOutMin=[]  DifferentiatorOutMax=[]  FilterDiffOutCoefMin=[]  FilterDiffOutCoefMax=[]  SumDenOutMin=[]  SumDenOutMax=[]  SumNumOutMin=[]  SumNumOutMax=[]  ReciprocalOutMin=[]  ReciprocalOutMax=[]  DivideOutMin=[]  DivideOutMax=[]  TunerSelectOption=Transfer Function Based (PID Tuner App)
  cfblk7 : simulink/Discrete/Difference  ICPrevInput=0.0  OutMin=[]  OutMax=[]  OutDataTypeStr=Inherit: Inherit via back propagation  OutDataType=fixdt(1, 16)  OutScaling=2^-10  DoSatur=off
  cfblk8 : DiscreteZeroPole  Poles=[0 0.5]  Gain=1  SampleTime=-1
  cfblk9 : DiscreteZeroPole  Poles=[0 0.5]  Gain=1  SampleTime=-1
  cyemi_{476..486} (11 alike) : DataTypeConversion  OutDataTypeStr=double
  cfblk2 : Outport
  cfblk14 : Outport  Port=2
  wires:
  cfblk9/1 -> cyemi_476/1
  cfblk8/1 -> cyemi_480/1
  cyemi_482/1 -> cfblk6/1
  cyemi_483/1 -> cfblk6/2
  cfblk7/1 -> cyemi_483/1
  cyemi_484/1 -> cfblk7/1
  cfblk1/1 -> cyemi_484/1
  cyemi_485/1 -> cfblk8/1
  cfblk13/1 -> cyemi_485/1
  cyemi_486/1 -> cfblk9/1
  cfblk6/1 -> cyemi_486/1
  cyemi_478/1 -> cyemi_481/1
  cyemi_479/1 -> cyemi_478/1, cfblk2/1
  cyemi_477/1 -> cfblk14/1
  cyemi_476/1 -> cyemi_479/1
  cyemi_481/1 -> cyemi_477/1
  cyemi_480/1 -> cyemi_482/1

== system sampleModel2432_pp_1_1_difftest/cfblk217 ==
  cfblk1 : Inport
  cfblk7 : Inport  Port=2
  Action Port : ActionPort  ActionType=then
  cfblk4 : Delay  DelayLengthSource=Input port
      settings: InputPortMap=u0,p1
  cfblk5 : Delay
  cfblk6 : DiscreteStateSpace  SampleTime=-1
  cyemi_{489..494} (6 alike) : DataTypeConversion  OutDataTypeStr=double
  cfblk2 : Outport
  wires:
  cfblk4/1 -> cyemi_490/1, cyemi_494/1
  cfblk6/1 -> cyemi_489/1
  cyemi_491/1 -> cfblk4/1
  cfblk5/1 -> cyemi_491/1
  cyemi_492/1 -> cfblk4/2
  cfblk1/1 -> cyemi_492/1
  cyemi_493/1 -> cfblk5/1
  cfblk7/1 -> cyemi_493/1
  cyemi_494/1 -> cfblk6/1
  cyemi_489/1 -> cfblk2/1

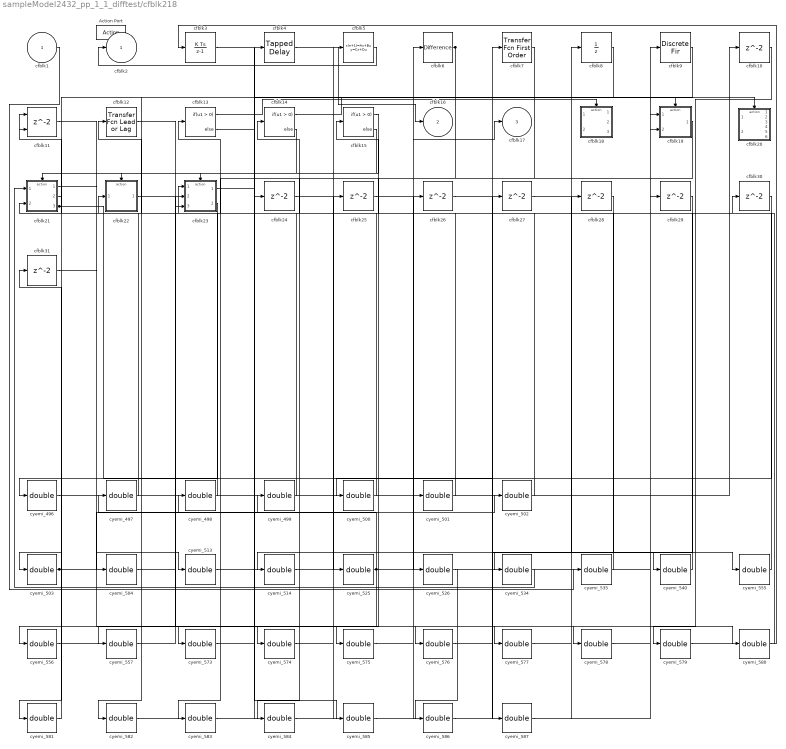
== system sampleModel2432_pp_1_1_difftest/cfblk218 ==
  cfblk1 : Inport
  Action Port : ActionPort  ActionType=else
  cfblk{10,24..31} (9 alike) : Delay
  cfblk11 : Delay  ShowEnablePort=on
      settings: InputPortMap=u0,e6
  cfblk12 : simulink/Discrete/Transfer Fcn Lead or Lag  PoleZ=0.95  ZeroZ=0.75  ICPrevOutput=0.0  ICPrevInput=0.0  DoSatur=off
      settings: SourceProductName=Simulink  SourceProductBaseCode=SL
  cfblk13 : If  SampleTime=1
  cfblk14 : If  SampleTime=1
  cfblk15 : If  SampleTime=1
  cfblk18 : Subsystem  TreatAsAtomicUnit=on
  cfblk19 : Subsystem  TreatAsAtomicUnit=on
  cfblk20 : Subsystem  TreatAsAtomicUnit=on
  cfblk21 : Subsystem  TreatAsAtomicUnit=on
  cfblk22 : Subsystem  TreatAsAtomicUnit=on
  cfblk23 : Subsystem  TreatAsAtomicUnit=on
  cfblk3 : DiscreteIntegrator  SampleTime=-1  ICPrevOutput=DiscIntNeverNeededParam  ICPrevScaledInput=DiscIntNeverNeededParam
  cfblk4 : simulink/Discrete/Tapped Delay  vinit=0.0  samptime=-1  NumDelays=1  DelayOrder=Oldest  includeCurrent=off
  cfblk5 : DiscreteStateSpace  SampleTime=-1
  cfblk6 : simulink/Discrete/Difference  ICPrevInput=0.0  OutMin=[]  OutMax=[]  OutDataTypeStr=Inherit: Inherit via back propagation  OutDataType=fixdt(1, 16)  OutScaling=2^-10  DoSatur=off
  cfblk7 : simulink/Discrete/Transfer Fcn First Order  PoleZ=0.95  ICPrevOutput=0.0  DoSatur=off
      settings: SourceProductName=Simulink
  cfblk8 : UnitDelay  SampleTime=-1
  cfblk9 : DiscreteFir
  cyemi_{496..504,513..514,525..526,534..535,540,555..557,573..587} (34 alike) : DataTypeConversion  OutDataTypeStr=double
  cfblk2 : Outport
  cfblk16 : Outport  Port=2
  cfblk17 : Outport  Port=3
  wires:
  cfblk4/1 -> cfblk16/1
  cfblk21/3(cfblk8) -> cyemi_526/1, cyemi_587/1
  cfblk5/1 -> cfblk2/1
  cfblk6/1 -> cyemi_557/1, cyemi_573/1
  cfblk13/1 -> cfblk18/Action
  cfblk13/2 -> cfblk19/Action
  cfblk14/1 -> cfblk20/Action
  cfblk14/2 -> cfblk21/Action
  cfblk15/1 -> cfblk22/Action
  cfblk15/2 -> cfblk23/Action
  cyemi_496/1 -> cfblk10/1
  cfblk23/2(cfblk14) -> cyemi_496/1
  cyemi_497/1 -> cfblk11/1
  cyemi_498/1 -> cfblk11/2
  cyemi_499/1 -> cfblk12/1
  cyemi_500/1 -> cfblk13/1
  cfblk30/1 -> cyemi_500/1
  cyemi_501/1 -> cfblk14/1
  cfblk25/1 -> cyemi_501/1
  cyemi_502/1 -> cfblk15/1
  cfblk21/2(cfblk7) -> cyemi_503/1
  cfblk31/1 -> cyemi_504/1
  cyemi_513/1 -> cfblk19/1(cfblk1)
  cfblk21/1(cfblk2) -> cyemi_513/1
  cyemi_514/1 -> cfblk19/2(cfblk10)
  cfblk29/1 -> cyemi_514/1
  cfblk24/1 -> cyemi_525/1
  cyemi_534/1 -> cfblk21/1(cfblk1)
  cfblk28/1 -> cyemi_534/1
  cyemi_535/1 -> cfblk21/2(cfblk6)
  cfblk1/1 -> cyemi_535/1
  cyemi_540/1 -> cfblk22/1(cfblk1)
  cfblk27/1 -> cyemi_540/1
  cyemi_555/1 -> cfblk23/1(cfblk1)
  cfblk26/1 -> cyemi_555/1
  cyemi_556/1 -> cfblk23/2(cfblk12)
  cyemi_557/1 -> cfblk23/3(cfblk13)
  cyemi_573/1 -> cfblk24/1
  cyemi_574/1 -> cfblk25/1
  cfblk22/1(cfblk2) -> cyemi_574/1
  cyemi_575/1 -> cfblk26/1
  cfblk7/1 -> cyemi_575/1
  cyemi_576/1 -> cfblk27/1
  cfblk3/1 -> cyemi_576/1
  cyemi_577/1 -> cfblk28/1
  cfblk12/1 -> cyemi_577/1
  cyemi_578/1 -> cfblk29/1
  cyemi_579/1 -> cfblk3/1
  cfblk10/1 -> cyemi_579/1
  cyemi_580/1 -> cfblk30/1
  cfblk11/1 -> cyemi_580/1
  cyemi_581/1 -> cfblk31/1
  cfblk8/1 -> cyemi_581/1
  cyemi_582/1 -> cfblk4/1
  cfblk9/1 -> cyemi_582/1
  cyemi_583/1 -> cfblk5/1
  cyemi_584/1 -> cfblk6/1
  cfblk19/1(cfblk2) -> cyemi_584/1
  cyemi_585/1 -> cfblk7/1
  cfblk23/1(cfblk2) -> cyemi_585/1
  cyemi_586/1 -> cfblk8/1
  cyemi_587/1 -> cfblk9/1
  cyemi_503/1 -> cyemi_502/1, cyemi_578/1
  cyemi_504/1 -> cyemi_499/1
  cyemi_525/1 -> cyemi_497/1, cfblk17/1, cyemi_583/1, cyemi_556/1, cyemi_498/1
  cyemi_526/1 -> cyemi_586/1

== system sampleModel2432_pp_1_1_difftest/cfblk219 ==
  cfblk1 : Inport
  cfblk8 : Inport  Port=2
  cfblk9 : Inport  Port=3
  Action Port : ActionPort  ActionType=then
  cfblk10 : Subsystem  TreatAsAtomicUnit=on
  cfblk11 : Subsystem  TreatAsAtomicUnit=on
  cfblk12 : Delay
  cfblk13 : Delay
  cfblk5 : simulink/Continuous/PID Controller  Controller=PID  TimeDomain=Discrete-time  SampleTime=-1  IntegratorMethod=Forward Euler  FilterMethod=Forward Euler  Form=Parallel  UseFilter=on  ControllerParametersSource=internal  P=1  I=1  D=0  N=100  InitialConditionSource=internal  InitialConditionForIntegrator=0  InitialConditionForFilter=0  ExternalReset=none  LimitOutput=off  UpperSaturationLimit=inf  LowerSaturationLimit=-inf  LinearizeAsGain=off  AntiWindupMode=none  Kb=1  TrackingMode=off  Kt=1  PParamMin=[]  PParamMax=[]  IParamMin=[]  IParamMax=[]  DParamMin=[]  DParamMax=[]  NParamMin=[]  NParamMax=[]  KbParamMin=[]  KbParamMax=[]  KtParamMin=[]  KtParamMax=[]  POutMin=[]  POutMax=[]  IOutMin=[]  IOutMax=[]  DOutMin=[]  DOutMax=[]  NOutMin=[]  NOutMax=[]  KbOutMin=[]  KbOutMax=[]  KtOutMin=[]  KtOutMax=[]  IntegratorOutMin=[]  IntegratorOutMax=[]  FilterOutMin=[]  FilterOutMax=[]  SumOutMin=[]  SumOutMax=[]  SumI1OutMin=[]  SumI1OutMax=[]  SumI2OutMin=[]  SumI2OutMax=[]  SumI3OutMin=[]  SumI3OutMax=[]  SumDOutMin=[]  SumDOutMax=[]  SaturationOutMin=[]  SaturationOutMax=[]  IntegratorContinuousStateAttributes=''  IntegratorStateMustResolveToSignalObject=off  IntegratorRTWStateStorageClass=Auto  FilterContinuousStateAttributes=''  FilterStateMustResolveToSignalObject=off  FilterRTWStateStorageClass=Auto  DifferentiatorICPrevScaledInput=0  DifferentiatorOutMin=[]  DifferentiatorOutMax=[]  FilterDiffOutCoefMin=[]  FilterDiffOutCoefMax=[]  SumDenOutMin=[]  SumDenOutMax=[]  SumNumOutMin=[]  SumNumOutMax=[]  ReciprocalOutMin=[]  ReciprocalOutMax=[]  DivideOutMin=[]  DivideOutMax=[]  TunerSelectOption=Transfer Function Based (PID Tuner App)
  cfblk6 : DiscreteFir
  cfblk7 : If  SampleTime=1
  cyemi_{591,606..608,613..619} (11 alike) : DataTypeConversion  OutDataTypeStr=double
  cfblk2 : Outport
  wires:
  cfblk7/1 -> cfblk10/Action
  cfblk7/2 -> cfblk11/Action
  cyemi_591/1 -> cfblk10/1(cfblk1)
  cfblk9/1 -> cyemi_591/1
  cyemi_606/1 -> cfblk11/1(cfblk1)
  cfblk1/1 -> cyemi_606/1
  cyemi_607/1 -> cfblk11/2(cfblk7)
  cfblk12/1 -> cyemi_607/1
  cyemi_608/1 -> cfblk11/3(cfblk8)
  cfblk5/1 -> cyemi_608/1
  cyemi_613/1 -> cfblk12/1
  cfblk10/1(cfblk2) -> cyemi_613/1
  cyemi_614/1 -> cfblk13/1
  cfblk11/1(cfblk2) -> cyemi_615/1
  cfblk6/1 -> cyemi_616/1
  cyemi_617/1 -> cfblk5/1
  cfblk8/1 -> cyemi_617/1
  cyemi_618/1 -> cfblk6/1
  cfblk11/2(cfblk9) -> cyemi_618/1
  cyemi_619/1 -> cfblk7/1
  cfblk13/1 -> cyemi_619/1
  cyemi_615/1 -> cyemi_614/1
  cyemi_616/1 -> cfblk2/1

== system sampleModel2432_pp_1_1_difftest/cfblk220 ==
  cfblk1 : Inport
  cfblk10 : Inport  Port=2
  cfblk11 : Inport  Port=3
  Action Port : ActionPort  ActionType=else
  cfblk3 : Delay
  cfblk4 : Delay  DelayLengthSource=Input port
      settings: InputPortMap=u0,p1
  cfblk5 : Delay  ShowEnablePort=on
      settings: InputPortMap=u0,e6
  cfblk6 : DiscreteIntegrator  SampleTime=-1  ICPrevOutput=DiscIntNeverNeededParam  ICPrevScaledInput=DiscIntNeverNeededParam
  cfblk7 : DiscreteTransferFcn
  cfblk8 : Delay  ShowEnablePort=on
      settings: InputPortMap=u0,e6
  cfblk9 : DiscreteStateSpace  SampleTime=-1
  cyemi_{624..633} (10 alike) : DataTypeConversion  OutDataTypeStr=double
  cfblk2 : Outport
  cfblk12 : Outport  Port=2
  cfblk13 : Outport  Port=3
  cfblk14 : Outport  Port=4
  wires:
  cfblk9/1 -> cfblk2/1, cyemi_631/1
  cfblk6/1 -> cyemi_624/1, cyemi_630/1
  cfblk5/1 -> cfblk14/1
  cfblk7/1 -> cfblk13/1
  cfblk11/1 -> cfblk12/1, cyemi_633/1
  cfblk3/1 -> cyemi_626/1, cyemi_632/1
  cyemi_624/1 -> cfblk3/1
  cyemi_625/1 -> cfblk4/1
  cfblk8/1 -> cyemi_625/1
  cyemi_626/1 -> cfblk4/2
  cyemi_627/1 -> cfblk5/1
  cfblk4/1 -> cyemi_627/1
  cyemi_628/1 -> cfblk5/2
  cfblk10/1 -> cyemi_628/1
  cyemi_629/1 -> cfblk6/1
  cfblk1/1 -> cyemi_629/1
  cyemi_630/1 -> cfblk7/1
  cyemi_631/1 -> cfblk8/1
  cyemi_632/1 -> cfblk8/2
  cyemi_633/1 -> cfblk9/1

== system sampleModel2432_pp_1_1_difftest/cfblk221 ==
  cfblk1 : Inport
  Action Port : ActionPort  ActionType=then
  cfblk3 : simulink/Discrete/Transfer Fcn Lead or Lag  PoleZ=0.95  ZeroZ=0.75  ICPrevOutput=0.0  ICPrevInput=0.0  DoSatur=off
      settings: SourceProductName=Simulink  SourceProductBaseCode=SL
  cfblk5 : DiscreteFir
  cfblk6 : Delay  ShowEnablePort=on
      settings: InputPortMap=u0,e6
  cfblk7 : DiscreteFilter
  cfblk8 : Delay
  cfblk9 : Delay
  cyemi_{635..642} (8 alike) : DataTypeConversion  OutDataTypeStr=double
  cfblk2 : Outport
  wires:
  cfblk7/1 -> cyemi_639/1, cyemi_641/1
  cfblk5/1 -> cfblk2/1
  cyemi_635/1 -> cfblk3/1
  cfblk8/1 -> cyemi_635/1
  cfblk6/1 -> cyemi_636/1
  cyemi_637/1 -> cfblk5/1
  cfblk1/1 -> cyemi_637/1
  cyemi_638/1 -> cfblk6/1
  cfblk9/1 -> cyemi_638/1
  cyemi_639/1 -> cfblk6/2
  cyemi_640/1 -> cfblk7/1
  cfblk3/1 -> cyemi_640/1
  cyemi_641/1 -> cfblk8/1
  cyemi_642/1 -> cfblk9/1
  cyemi_636/1 -> cyemi_642/1

== system sampleModel2432_pp_1_1_difftest/cfblk222 ==
  cfblk1 : Inport
  cfblk6 : Inport  Port=2
  cfblk7 : Inport  Port=3
  Action Port : ActionPort  ActionType=else
  cfblk3 : simulink/Discrete/Transfer Fcn Lead or Lag  PoleZ=0.95  ZeroZ=0.75  ICPrevOutput=0.0  ICPrevInput=0.0  DoSatur=off
      settings: SourceProductName=Simulink  SourceProductBaseCode=SL
  cfblk4 : Delay  ShowEnablePort=on
      settings: InputPortMap=u0,e6
  cfblk5 : DiscreteFilter
  cyemi_{646..649} (4 alike) : DataTypeConversion  OutDataTypeStr=double
  cfblk2 : Outport
  cfblk8 : Outport  Port=2
  wires:
  cfblk4/1 -> cfblk8/1
  cfblk1/1 -> cfblk2/1
  cyemi_646/1 -> cfblk3/1
  cfblk6/1 -> cyemi_646/1
  cyemi_647/1 -> cfblk4/1
  cfblk7/1 -> cyemi_647/1
  cyemi_648/1 -> cfblk4/2
  cfblk5/1 -> cyemi_648/1
  cyemi_649/1 -> cfblk5/1
  cfblk3/1 -> cyemi_649/1

== system sampleModel2432_pp_1_1_difftest/cfblk223 ==
  cfblk1 : Inport
  cfblk8 : Inport  Port=2
  Action Port : ActionPort  ActionType=then
  cfblk3 : Delay  DelayLengthSource=Input port
      settings: InputPortMap=u0,p1
  cfblk4 : DiscreteFilter
  cfblk5 : DiscreteZeroPole  Poles=[0 0.5]  Gain=1  SampleTime=-1
  cfblk6 : DiscreteStateSpace  SampleTime=-1
  cfblk7 : simulink/Discrete/Difference  ICPrevInput=0.0  OutMin=[]  OutMax=[]  OutDataTypeStr=Inherit: Inherit via back propagation  OutDataType=fixdt(1, 16)  OutScaling=2^-10  DoSatur=off
  cyemi_{652..657} (6 alike) : DataTypeConversion  OutDataTypeStr=double
  cfblk2 : Outport
  cfblk9 : Outport  Port=2
  wires:
  cfblk8/1 -> cfblk2/1
  cfblk6/1 -> cyemi_653/1, cyemi_654/1
  cfblk3/1 -> cfblk9/1
  cyemi_652/1 -> cfblk3/1
  cfblk4/1 -> cyemi_652/1
  cyemi_653/1 -> cfblk3/2
  cyemi_654/1 -> cfblk4/1
  cyemi_655/1 -> cfblk5/1
  cfblk7/1 -> cyemi_655/1
  cyemi_656/1 -> cfblk6/1
  cfblk5/1 -> cyemi_656/1
  cyemi_657/1 -> cfblk7/1
  cfblk1/1 -> cyemi_657/1

== system sampleModel2432_pp_1_1_difftest/cfblk224 ==
  cfblk1 : Inport
  Action Port : ActionPort  ActionType=else
  cfblk{10..13} (4 alike) : Delay
  cfblk3 : simulink/Discrete/Difference  ICPrevInput=0.0  OutMin=[]  OutMax=[]  OutDataTypeStr=Inherit: Inherit via back propagation  OutDataType=fixdt(1, 16)  OutScaling=2^-10  DoSatur=off
  cfblk6 : Delay  DelayLengthSource=Input port
      settings: InputPortMap=u0,p1
  cfblk8 : Subsystem  TreatAsAtomicUnit=on
  cfblk9 : Subsystem  TreatAsAtomicUnit=on
  cyemi_{659..671,685..686} (15 alike) : DataTypeConversion  OutDataTypeStr=double
  cfblk2 : Outport
  wires:
  cfblk9/1(cfblk2) -> cfblk2/1
  cfblk6/1 -> cyemi_661/1, cyemi_665/1
  cyemi_659/1 -> cfblk10/1
  cyemi_660/1 -> cfblk11/1
  cyemi_661/1 -> cfblk12/1
  cyemi_662/1 -> cfblk13/1
  cfblk8/4(cfblk16) -> cyemi_662/1
  cyemi_663/1 -> cfblk3/1
  cfblk8/1(cfblk2) -> cyemi_663/1
  cfblk3/1 -> cyemi_664/1
  cyemi_666/1 -> cfblk6/1
  cfblk9/2(cfblk9) -> cyemi_666/1
  cyemi_667/1 -> cfblk6/2
  cfblk8/3(cfblk15) -> cyemi_667/1
  cfblk13/1 -> cyemi_668/1
  cyemi_669/1 -> cfblk8/1(cfblk1)
  cfblk10/1 -> cyemi_669/1
  cyemi_670/1 -> cfblk8/2(cfblk12)
  cfblk1/1 -> cyemi_670/1
  cyemi_671/1 -> cfblk8/3(cfblk13)
  cfblk12/1 -> cyemi_671/1
  cyemi_685/1 -> cfblk9/1(cfblk1)
  cfblk11/1 -> cyemi_685/1
  cyemi_686/1 -> cfblk9/2(cfblk8)
  cfblk8/2(cfblk14) -> cyemi_686/1
  cyemi_665/1 -> cyemi_660/1
  cyemi_664/1 -> cyemi_659/1
